simulink model "sfcndemo_port_constant"  (Simulink 7.6)
settings: Solver=FixedStepDiscrete  StartTime=0.0  StopTime=10  RelTol=1e-3
Description:
  | Port-Based Sample Time C-MEX S-function Including Constant Sample Time
settings Model: Creator=The MathWorks Inc.  ExtModeAutoUpdateStatusClock=off
settings OptimizationCC: BooleanDataType=off  InlineParams=on  InlineInvariantSignals=on  InitFltsAndDblsToZero=on
settings DebuggingCC: SaveWithParameterizedLinksMsg=none  SignalResolutionControl=TryResolveAllWithWarning  SolverPrmCheckMsg=none  MultiTaskDSMMsg=warning  MultiTaskCondExecSysMsg=none
settings HardwareCC: TargetUnknown=on
settings RTWCC: IncludeERTFirstTime=on
settings CodeAppCC: CustomSymbolStrFcn=$F$N$M
settings GRTTargetCC: TargetFcnLib=ansi_tfl_tmw.mat

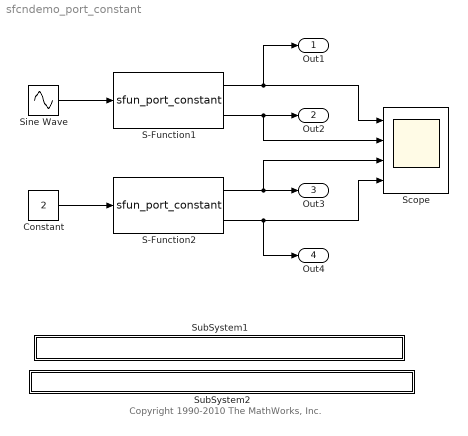
== system sfcndemo_port_constant ==
  note: Copyright 1990-2010 The MathWorks, Inc.
  Constant : Constant  Value=2
  S-Function1 : S-Function  FunctionName=sfun_port_constant  Parameters=5  EnableBusSupport=off
  S-Function2 : S-Function  FunctionName=sfun_port_constant  Parameters=7  EnableBusSupport=off
  Scope : Scope  NumInputPorts=4
      settings: TimeRange=10  YMin=-5~4~13~6  YMax=5~6~15~8
  Sine Wave : Sin  SampleTime=0
  SubSystem1 : Subsystem  mask{filename=sfun_port_constant.c}
      mask init:
      | x=sfundemo_maskdisp;
      settings: AttributesFormatString=\n  OpenFcn=sfundemo_openfcn
      mask Display: disp(x);
  SubSystem2 : Subsystem  mask{filename=sfun_port_constant.tlc}
      mask init:
      | x=sfundemo_maskdisp;
      settings: AttributesFormatString=\n  OpenFcn=sfundemo_openfcn
      mask Display: disp(x);
  Out1 : Outport
  Out2 : Outport  Port=2
  Out3 : Outport  Port=3
  Out4 : Outport  Port=4
  wires:
  Sine Wave/1 -> S-Function1/1
  S-Function1/1 -> Out1/1, Scope/1
  S-Function1/2 -> Out2/1, Scope/2
  Constant/1 -> S-Function2/1
  S-Function2/1 -> Out3/1, Scope/3
  S-Function2/2 -> Scope/4, Out4/1

== system sfcndemo_port_constant/SubSystem1 ==

== system sfcndemo_port_constant/SubSystem2 ==
